simulink model "cruise_control"  (R2020b)
settings: Solver=VariableStepAuto  StartTime=0.0  StopTime=10.0  RelTol=1e-3
values from neighbouring files (symbols this model uses):
  b = 50.0    [parameter_data.sldd]
  Kp = 1000.0    [parameter_data.sldd]
  m = 1000.0    [parameter_data.sldd]
undefined symbols (not defined in the file or in its folder): Ks
settings Model: Creator=Vrunda M Balgi  LastModifiedBy=Vrunda M Balgi

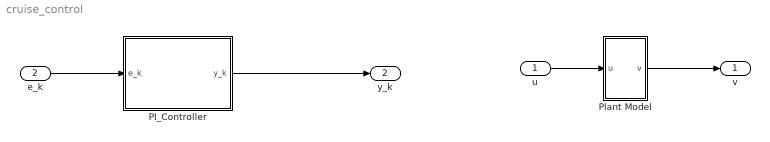
== system cruise_control ==
  u : Inport
  e_k : Inport  Port=2
  PI_Controller : Subsystem
  Plant Model : Subsystem
  v : Outport
  y_k : Outport  Port=2
  wires:
  u/1 -> Plant Model/1(u)
  Plant Model/1(v) -> v/1
  e_k/1 -> PI_Controller/1(e_k)
  PI_Controller/1(y_k) -> y_k/1

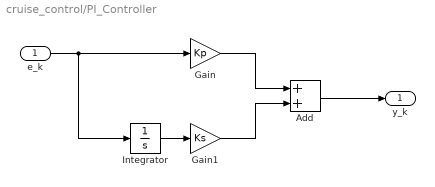
== system cruise_control/PI_Controller ==
  e_k : Inport
  Add : Sum
  Gain : Gain  Gain=Kp
  Gain1 : Gain  Gain=Ks
  Integrator : Integrator
  y_k : Outport
  wires:
  e_k/1 -> Integrator/1, Gain/1
  Gain/1 -> Add/1
  Gain1/1 -> Add/2
  Integrator/1 -> Gain1/1
  Add/1 -> y_k/1

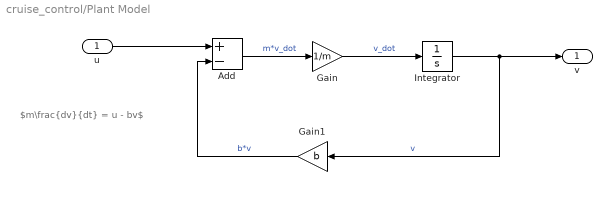
== system cruise_control/Plant Model ==
  note: $m\frac{dv}{dt} = u - bv$
  u : Inport
  Add : Sum  Inputs=+-
  Gain : Gain  Gain=1/m
  Gain1 : Gain  Gain=b
  Integrator : Integrator
  v : Outport
  wires:
  Integrator/1 -> v/1, Gain1/1  "v"
  Add/1 -> Gain/1  "m*v_dot"
  u/1 -> Add/1
  Gain1/1 -> Add/2  "b*v"
  Gain/1 -> Integrator/1  "v_dot"
